simulink model "VIM"  (R2022b)
settings: Solver=ode45  StartTime=0.0  StopTime=1  RelTol=1e-3
PreLoadFcn:
  | % Define motor parameters
  | params.Rs = 0.435;
  | params.Rr = 0.816;
  | params.Ls = 0.006;
  | params.Lr = 0.006;
  | params.Lm = 0.006;
  | params.Xls = 0.006;
  | params.Xlr = 0.006;
  | params.omega_r = 314;
  | params.omega_s = 314;
  | params.dt = 1e-4;
model workspace (MAT data in the model file):
  Lm = Simulink.Parameter
  Lm.Value = 0.006
  Lm.DataType = 'auto'
  Lm.Complexity = 'real'
  Lm.Dimensions = [1 1]
  Lr = Simulink.Parameter
  Lr.Value = 0.006
  Lr.DataType = 'auto'
  Lr.Complexity = 'real'
  Lr.Dimensions = [1 1]
  Ls = Simulink.Parameter
  Ls.Value = 0.006
  Ls.DataType = 'auto'
  Ls.Complexity = 'real'
  Ls.Dimensions = [1 1]
  Rr = Simulink.Parameter
  Rr.Value = 0.816
  Rr.DataType = 'auto'
  Rr.Complexity = 'real'
  Rr.Dimensions = [1 1]
  Rs = Simulink.Parameter
  Rs.Value = 0.435
  Rs.DataType = 'auto'
  Rs.Complexity = 'real'
  Rs.Dimensions = [1 1]
  Sig = Simulink.Signal
  Sig.DataType = 'auto'
  Sig.Dimensions = -1
  Sig.DimensionsMode = 'auto'
  Sig.Complexity = 'auto'
  Sig.SampleTime = -1
  Sig.SamplingMode = 'auto'
  Xlr = Simulink.Parameter
  Xlr.Value = 0.006
  Xlr.DataType = 'auto'
  Xlr.Complexity = 'real'
  Xlr.Dimensions = [1 1]
  Xls = Simulink.Parameter
  Xls.Value = 0.006
  Xls.DataType = 'auto'
  Xls.Complexity = 'real'
  Xls.Dimensions = [1 1]
  dt = Simulink.Parameter
  dt.Value = 0.0001
  dt.DataType = 'auto'
  dt.Complexity = 'real'
  dt.Dimensions = [1 1]
  omega_r = Simulink.Parameter
  omega_r.Value = 314
  omega_r.DataType = 'auto'
  omega_r.Complexity = 'real'
  omega_r.Dimensions = [1 1]
  omega_s = Simulink.Parameter
  omega_s.Value = 314
  omega_s.DataType = 'auto'
  omega_s.Complexity = 'real'
  omega_s.Dimensions = [1 1]
undefined symbols (not defined in the file or in its folder): D1, lagging, motorParams, params_struct_torque, pulse
libraries: slpidlib x4, spsabctodq0Lib x4, spsPLL3phLib x1, spsPulseGeneratorThyristor6PulseLib x1, spsdq0toabcLib x1, spspowerguiLib x1
settings Model: Creator=Dong  LastModifiedBy=Dong

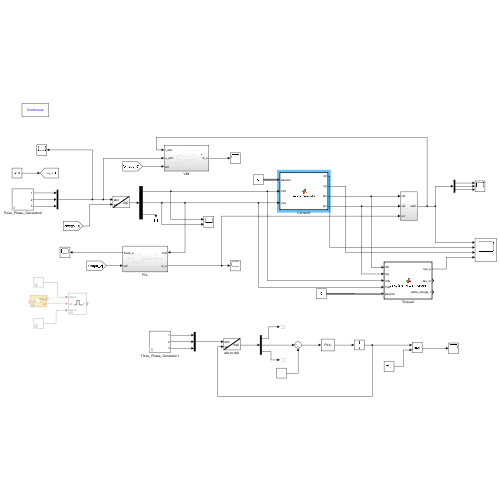
[thumbnail: Simulink's stored preview of the top-level diagram]
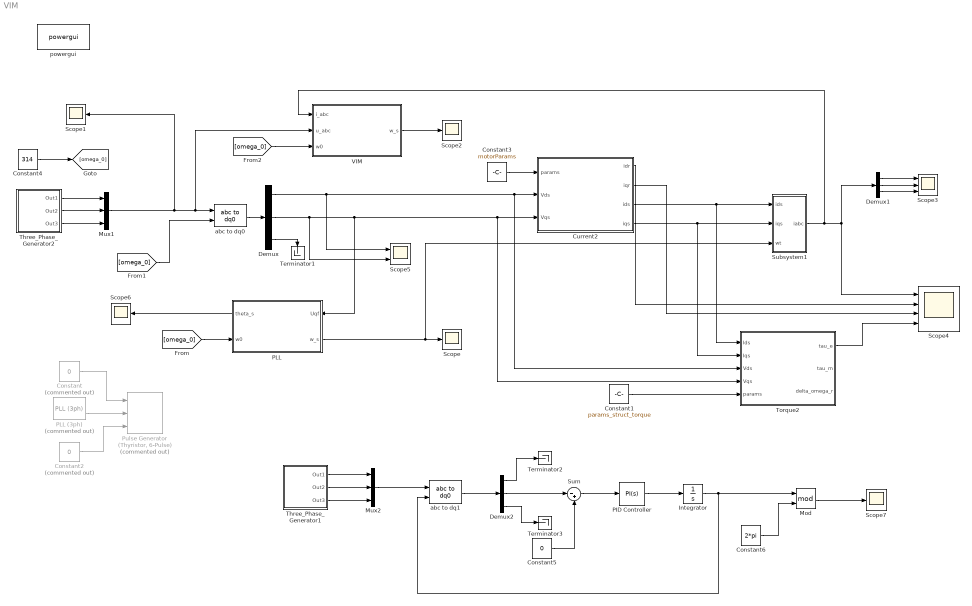
== system VIM ==
  Constant : Constant  Commented=on  Value=0
  Constant1 : Constant  Value=params_struct_torque  OutDataTypeStr=Bus: paramsBusTorque
  Constant2 : Constant  Commented=on  Value=0
  Constant3 : Constant  Value=motorParams  OutDataTypeStr=Bus: motorParamsBus
  Constant4 : Constant  Value=314
  Constant5 : Constant  Value=0
  Constant6 : Constant  Value=2*pi
  Current2 : MATLAB Function  TreatAsAtomicUnit=on
  Demux : Demux  Outputs=3
  Demux1 : Demux  Outputs=3
  Demux2 : Demux  Outputs=3
  Integrator : Integrator
  Mod : Math  Operator=mod
  Mux1 : Mux  Inputs=3
  Mux2 : Mux  Inputs=3
  PID Controller : slpidlib/PID Controller  Controller=PI  Form=Parallel  TimeDomain=Continuous-time  UseExternalTs=off  SampleTime=-1  IntegratorMethod=Forward Euler  FilterMethod=Forward Euler  ControllerParametersSource=internal  P=70  I=2500  UseKiTs=off  D=0  N=100  UseFilter=on  TunerSelectOption=Transfer Function Based (PID Tuner App)  InitialConditionSource=internal  InitialConditionForIntegrator=0  InitialConditionForFilter=0  DifferentiatorICPrevScaledInput=0  ExternalReset=none  TrackingMode=off  Kt=1  LimitOutput=off  SatLimitsSource=internal  UpperSaturationLimit=inf  LowerSaturationLimit=-inf  LinearizeAsGain=on  AntiWindupMode=none  Kb=1  LimitIntegrator=off  UpperIntegratorSaturationLimit=inf  LowerIntegratorSaturationLimit=-inf  POutMin=[]  POutMax=[]  IOutMin=[]  IOutMax=[]  DOutMin=[]  DOutMax=[]  NOutMin=[]  NOutMax=[]  SumOutMin=[]  SumOutMax=[]  SaturationOutMin=[]  SaturationOutMax=[]  PParamMin=[]  PParamMax=[]  IParamMin=[]  IParamMax=[]  DParamMin=[]  DParamMax=[]  NParamMin=[]  NParamMax=[]  KbParamMin=[]  KbParamMax=[]  KtParamMin=[]  KtParamMax=[]  KbOutMin=[]  KbOutMax=[]  KtOutMin=[]  KtOutMax=[]  IntegratorOutMin=[]  IntegratorOutMax=[]  FilterOutMin=[]  FilterOutMax=[]  SumI1OutMin=[]  SumI1OutMax=[]  SumI2OutMin=[]  SumI2OutMax=[]  SumI3OutMin=[]  SumI3OutMax=[]  SumI4OutMin=[]  SumI4OutMax=[]  SumDOutMin=[]  SumDOutMax=[]  DifferentiatorOutMin=[]  DifferentiatorOutMax=[]  FilterDiffOutCoefMin=[]  FilterDiffOutCoefMax=[]  ReciprocalOutMin=[]  ReciprocalOutMax=[]  SumDenOutMin=[]  SumDenOutMax=[]  SumNumOutMin=[]  SumNumOutMax=[]  DivideOutMin=[]  DivideOutMax=[]  UdiffTsProdOutMin=[]  UdiffTsProdOutMax=[]  NTsProdOutMin=[]  NTsProdOutMax=[]  UintegralTsProdOutMin=[]  UintegralTsProdOutMax=[]  UngainTsProdOutMin=[]  UngainTsProdOutMax=[]  ClampingZeroOutDataTypeStr=Inherit: Inherit via back propagation  ClampingZeroOutMin=[]  ClampingZeroOutMax=[]  FilterDenConstantOutDataTypeStr=Inherit: Inherit via back propagation  FilterDenConstantOutMin=[]  FilterDenConstantOutMax=[]  PCopyOutDataTypeStr=Inherit: Inherit via back propagation  PCopyOutMin=[]  PCopyOutMax=[]  NCopyOutDataTypeStr=Inherit: Inherit via back propagation  NCopyOutMin=[]  NCopyOutMax=[]  IntegratorContinuousStateAttributes=''  IntegratorStateMustResolveToSignalObject=off  IntegratorRTWStateStorageClass=Auto  FilterContinuousStateAttributes=''  FilterStateMustResolveToSignalObject=off  FilterRTWStateStorageClass=Auto  ParallelPVariant=InternalParameters  IdealPVariant=Disabled  IVariant=InternalParameters  DVariant=Disabled  IntegratorVariant=Continuous  SatVariant=Disabled  AWVariant=Passthrough  PCopyVariant=Disabled  TRVariant=Disabled  FdbkBlocksVariant=Forward  IdealPFdbkVariant=Disabled  SatFdbkVariant=Disabled  DerivativeFilterVariant=Disabled  NVariant=Disabled  NCopyVariant=Disabled_SignalSpec  FilterICVariant=Disabled  IntegratorICVariant=InternalICs  ExternalResetVariant=Disabled  TRSumVariant=Passthrough  SumFdbkVariant=Disabled  SumVariant=Sum_PI  TsampFilterVariant=InternalTs  TsampNgainVariant=Passthrough  TsampIntegralVariant=Passthrough  ExternalSaturationOutDataTypeStr=Inherit: Same as second input
  PLL : Subsystem
      settings: PortSchema="{\"entries\":[{\"content\":{\"sides\":[{\"content\":{\"connectorIds\":[\"Out2\",\"In1\"]},\"type\":\"ConnectorPlacement.EquallySpacedRectSide\",\"uuid\":\"af5f83a4-7527-4799-92d3-33395b605044\"},{\"content\":{\"connectorIds\":[\"In2\",\"Out1\"],\"side\":\"RIGHT\"},\"type\":\"ConnectorPlacement.EquallySpacedRectSide\",\"uuid\":\"36de21ae-8d82-4c7b-9387-ed93b71e64bb\"},{\"content\":{\"connectorIds\":[],\"side\":\"TOP\"},\"type\":\"ConnectorPlacement.EquallySpacedRectSide\",\"uuid\":\"440d0f6f-e820-4256-be94-60c050b455d0\"}]},\"type\":\"ConnectorPlacement.EquallySpacedConnector\",\"uuid\":\"20572b40-4a5f-41c5-8c6b-bc5bfa0c4be0\"}],\"packageUris\":[\"http://schema.mathworks.com/mf0/Connector/R2020b\"],\"version\":\"1.0\"}"
  PLL (3ph) : spsPLL3phLib/PLL (3ph)  Commented=on  Fmin=49  Par_Init=[0, 50]  ParK=[180, 3200, 1]  TcD=1e-4  MaxRateChangeFreq=12  FilterCutOffFreq=25  Ts=0  AGC=on
  "Pulse Generator (Thyristor, 6-Pulse)" : spsPulseGeneratorThyristor6PulseLib/Pulse Generator (Thyristor, 6-Pulse)  Commented=on  GenType=6-pulse  Delta=D1 (lagging)  pwidth=60  Double_Pulse=off  Ts=0
      settings: LibrarySourceBlock=|
      | sps_lib/Power Electronics/Power Electronics Control/Pulse Generator
      | (Thyristor, 6-Pulse)
  Scope{,1..2,6..7} (5 alike) : Scope
  Scope3 : Scope  NumInputPorts=3
  Scope4 : Scope  NumInputPorts=4
  Scope5 : Scope  NumInputPorts=2
  Subsystem1 : Subsystem
  Sum : Sum  Inputs=|-+
  Terminator1 : Terminator
  Terminator2 : Terminator
  Terminator3 : Terminator
  Three_Phase_Generator1 : Subsystem  mask{freq=50, alpha=120, amplitude=240}
      mask prompts: freq "Frequenz"; alpha "Pahse"
      mask DialogControl ParameterGroupVar Prompt: 参数
  Three_Phase_Generator2 : Subsystem  mask{freq=50, alpha=120, amplitude=240}
      mask prompts: freq "Frequenz"; alpha "Pahse"
      mask DialogControl ParameterGroupVar Prompt: 参数
  Torque2 : MATLAB Function  TreatAsAtomicUnit=on
  VIM : Subsystem
  abc to dq0 : spsabctodq0Lib/abc to dq0  Alignment=90 degrees behind phase A axis
  abc to dq1 : spsabctodq0Lib/abc to dq0  Alignment=90 degrees behind phase A axis
  powergui : spspowerguiLib/powergui  Priority=1  SimulationMode=Continuous  SampleTime=50e-6  frequency=60  Iterations=50  frequencyindice=60  Pbase=100e6  ErrMax=1e-4  UnitsV=kV  UnitsW=MW  buscounter=0  FunctionMessages=off  echomessages=off  EnableUseOfTLC=off  CurrentSourceSwitches=off  DisableSnubberDevices=off  DisableRonSwitches=off  DisableVfSwitches=off  DisplayEquations=off  AutomaticDiscreteSolvers=off  SolverType=Tustin/Backward Euler (TBE)  Interpol=off  ExternalGateDelay=off  methode=off  Ts=100  x0status=blocks  SPID=on  SwTol=0  HookPort=off  NonlinearTolerance=1e-4  nMaxIteration=100  ContinueOnMaxIteration=off  RestoreLinks=warning  ResistiveCurrentMeasurement=off  Frange=[0:2:500]  Ylog=off  Xlog=on  ShowGrid=off  save=off  variable=ZData  structure=0  ZoomFFT=off  StartTime=0.0  cycles=1  DisplayStyle=1  fundamental=60  FreqAxis=off  MaxFrequency=1000  frequencyindicesteady=1  RmsSteady=1  display=off
  wires:
  Mux1/1 -> Scope1/1, abc to dq0/1, VIM/2(u_abc)
  abc to dq0/1 -> Demux/1
  Constant1/1 -> Torque2/5(params)
  Constant3/1 -> Current2/1(params)
  Demux/3 -> Terminator1/1
  Current2/3(ids) -> Torque2/1(Ids), Subsystem1/1(ids)
  Current2/4(iqs) -> Torque2/2(Iqs), Subsystem1/2(iqs)
  Demux/1 -> Scope5/1, Current2/2(Vds), Torque2/3(Vds)
  PLL/1(w_s) -> Scope/1, Subsystem1/3(wt)
  VIM/1(w_s) -> Scope2/1
  Torque2/1(tau_e) -> Scope4/4
  Current2/2(iqr) -> Scope4/3
  Current2/1(idr) -> Scope4/2
  Subsystem1/1(iabc) -> VIM/1(i_abc), Scope4/1, Demux1/1
  Demux/2 -> Scope5/2, Torque2/4(Vqs), Current2/3(Vqs), PLL/2(Uqf)
  Demux1/1 -> Scope3/1
  Demux1/2 -> Scope3/2
  Demux1/3 -> Scope3/3
  Three_Phase_Generator2/1(Out1) -> Mux1/1
  Three_Phase_Generator2/2(Out2) -> Mux1/2
  Three_Phase_Generator2/3(Out3) -> Mux1/3
  Constant4/1 -> [omega_0]
  [omega_0] -> PLL/1(w0)
  PLL/2(theta_s) -> Scope6/1
  [omega_0] -> VIM/3(w0)
  [omega_0] -> abc to dq0/2
  PLL (3ph)/2 -> "Pulse Generator (Thyristor, 6-Pulse)"/2
  Constant/1 -> "Pulse Generator (Thyristor, 6-Pulse)"/1
  Constant2/1 -> "Pulse Generator (Thyristor, 6-Pulse)"/3
  Three_Phase_Generator1/3(Out3) -> Mux2/3
  Three_Phase_Generator1/2(Out2) -> Mux2/2
  Three_Phase_Generator1/1(Out1) -> Mux2/1
  Mux2/1 -> abc to dq1/1
  abc to dq1/1 -> Demux2/1
  Demux2/1 -> Terminator2/1
  Demux2/3 -> Terminator3/1
  Constant5/1 -> Sum/2
  Sum/1 -> PID Controller/1
  PID Controller/1 -> Integrator/1
  Integrator/1 -> Mod/1, abc to dq1/2
  Demux2/2 -> Sum/1
  Constant6/1 -> Mod/2
  Mod/1 -> Scope7/1

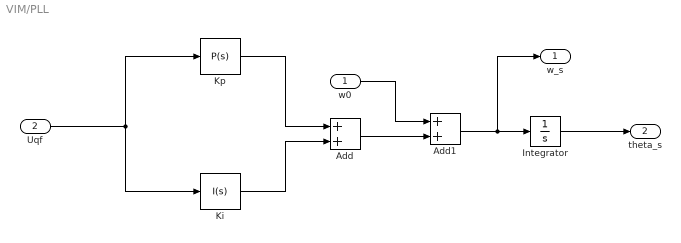
== system VIM/PLL ==
  w0 : Inport
  Uqf : Inport  Port=2
  Add : Sum
  Add1 : Sum
  Integrator : Integrator
  Ki : slpidlib/PID Controller  Controller=I  Form=Parallel  TimeDomain=Continuous-time  UseExternalTs=off  SampleTime=-1  IntegratorMethod=Forward Euler  FilterMethod=Forward Euler  ControllerParametersSource=internal  P=1  I=5  UseKiTs=off  D=0  N=100  UseFilter=on  TunerSelectOption=Transfer Function Based (PID Tuner App)  InitialConditionSource=internal  InitialConditionForIntegrator=0  InitialConditionForFilter=0  DifferentiatorICPrevScaledInput=0  ExternalReset=none  TrackingMode=off  Kt=1  LimitOutput=off  SatLimitsSource=internal  UpperSaturationLimit=inf  LowerSaturationLimit=-inf  LinearizeAsGain=on  AntiWindupMode=none  Kb=1  LimitIntegrator=off  UpperIntegratorSaturationLimit=inf  LowerIntegratorSaturationLimit=-inf  POutMin=[]  POutMax=[]  IOutMin=[]  IOutMax=[]  DOutMin=[]  DOutMax=[]  NOutMin=[]  NOutMax=[]  SumOutMin=[]  SumOutMax=[]  SaturationOutMin=[]  SaturationOutMax=[]  PParamMin=[]  PParamMax=[]  IParamMin=[]  IParamMax=[]  DParamMin=[]  DParamMax=[]  NParamMin=[]  NParamMax=[]  KbParamMin=[]  KbParamMax=[]  KtParamMin=[]  KtParamMax=[]  KbOutMin=[]  KbOutMax=[]  KtOutMin=[]  KtOutMax=[]  IntegratorOutMin=[]  IntegratorOutMax=[]  FilterOutMin=[]  FilterOutMax=[]  SumI1OutMin=[]  SumI1OutMax=[]  SumI2OutMin=[]  SumI2OutMax=[]  SumI3OutMin=[]  SumI3OutMax=[]  SumI4OutMin=[]  SumI4OutMax=[]  SumDOutMin=[]  SumDOutMax=[]  DifferentiatorOutMin=[]  DifferentiatorOutMax=[]  FilterDiffOutCoefMin=[]  FilterDiffOutCoefMax=[]  ReciprocalOutMin=[]  ReciprocalOutMax=[]  SumDenOutMin=[]  SumDenOutMax=[]  SumNumOutMin=[]  SumNumOutMax=[]  DivideOutMin=[]  DivideOutMax=[]  UdiffTsProdOutMin=[]  UdiffTsProdOutMax=[]  NTsProdOutMin=[]  NTsProdOutMax=[]  UintegralTsProdOutMin=[]  UintegralTsProdOutMax=[]  UngainTsProdOutMin=[]  UngainTsProdOutMax=[]  ClampingZeroOutDataTypeStr=Inherit: Inherit via back propagation  ClampingZeroOutMin=[]  ClampingZeroOutMax=[]  FilterDenConstantOutDataTypeStr=Inherit: Inherit via back propagation  FilterDenConstantOutMin=[]  FilterDenConstantOutMax=[]  PCopyOutDataTypeStr=Inherit: Inherit via back propagation  PCopyOutMin=[]  PCopyOutMax=[]  NCopyOutDataTypeStr=Inherit: Inherit via back propagation  NCopyOutMin=[]  NCopyOutMax=[]  IntegratorContinuousStateAttributes=''  IntegratorStateMustResolveToSignalObject=off  IntegratorRTWStateStorageClass=Auto  FilterContinuousStateAttributes=''  FilterStateMustResolveToSignalObject=off  FilterRTWStateStorageClass=Auto  ParallelPVariant=Disabled  IdealPVariant=Disabled  IVariant=InternalParameters  DVariant=Disabled  IntegratorVariant=Continuous  SatVariant=Disabled  AWVariant=Passthrough  PCopyVariant=Disabled  TRVariant=Disabled  FdbkBlocksVariant=Forward  IdealPFdbkVariant=Disabled  SatFdbkVariant=Disabled  DerivativeFilterVariant=Disabled  NVariant=Disabled  NCopyVariant=Disabled_SignalSpec  FilterICVariant=Disabled  IntegratorICVariant=InternalICs  ExternalResetVariant=Disabled  TRSumVariant=Passthrough  SumFdbkVariant=Disabled  SumVariant=Passthrough_I  TsampFilterVariant=InternalTs  TsampNgainVariant=Passthrough  TsampIntegralVariant=Passthrough  ExternalSaturationOutDataTypeStr=Inherit: Same as second input
  Kp : slpidlib/PID Controller  Controller=P  Form=Parallel  TimeDomain=Continuous-time  UseExternalTs=off  SampleTime=-1  IntegratorMethod=Forward Euler  FilterMethod=Forward Euler  ControllerParametersSource=internal  P=7  I=1  UseKiTs=off  D=0  N=100  UseFilter=on  TunerSelectOption=Transfer Function Based (PID Tuner App)  InitialConditionSource=internal  InitialConditionForIntegrator=0  InitialConditionForFilter=0  DifferentiatorICPrevScaledInput=0  ExternalReset=none  TrackingMode=off  Kt=1  LimitOutput=off  SatLimitsSource=internal  UpperSaturationLimit=inf  LowerSaturationLimit=-inf  LinearizeAsGain=on  AntiWindupMode=none  Kb=1  LimitIntegrator=off  UpperIntegratorSaturationLimit=inf  LowerIntegratorSaturationLimit=-inf  POutMin=[]  POutMax=[]  IOutMin=[]  IOutMax=[]  DOutMin=[]  DOutMax=[]  NOutMin=[]  NOutMax=[]  SumOutMin=[]  SumOutMax=[]  SaturationOutMin=[]  SaturationOutMax=[]  PParamMin=[]  PParamMax=[]  IParamMin=[]  IParamMax=[]  DParamMin=[]  DParamMax=[]  NParamMin=[]  NParamMax=[]  KbParamMin=[]  KbParamMax=[]  KtParamMin=[]  KtParamMax=[]  KbOutMin=[]  KbOutMax=[]  KtOutMin=[]  KtOutMax=[]  IntegratorOutMin=[]  IntegratorOutMax=[]  FilterOutMin=[]  FilterOutMax=[]  SumI1OutMin=[]  SumI1OutMax=[]  SumI2OutMin=[]  SumI2OutMax=[]  SumI3OutMin=[]  SumI3OutMax=[]  SumI4OutMin=[]  SumI4OutMax=[]  SumDOutMin=[]  SumDOutMax=[]  DifferentiatorOutMin=[]  DifferentiatorOutMax=[]  FilterDiffOutCoefMin=[]  FilterDiffOutCoefMax=[]  ReciprocalOutMin=[]  ReciprocalOutMax=[]  SumDenOutMin=[]  SumDenOutMax=[]  SumNumOutMin=[]  SumNumOutMax=[]  DivideOutMin=[]  DivideOutMax=[]  UdiffTsProdOutMin=[]  UdiffTsProdOutMax=[]  NTsProdOutMin=[]  NTsProdOutMax=[]  UintegralTsProdOutMin=[]  UintegralTsProdOutMax=[]  UngainTsProdOutMin=[]  UngainTsProdOutMax=[]  ClampingZeroOutDataTypeStr=Inherit: Inherit via back propagation  ClampingZeroOutMin=[]  ClampingZeroOutMax=[]  FilterDenConstantOutDataTypeStr=Inherit: Inherit via back propagation  FilterDenConstantOutMin=[]  FilterDenConstantOutMax=[]  PCopyOutDataTypeStr=Inherit: Inherit via back propagation  PCopyOutMin=[]  PCopyOutMax=[]  NCopyOutDataTypeStr=Inherit: Inherit via back propagation  NCopyOutMin=[]  NCopyOutMax=[]  IntegratorContinuousStateAttributes=''  IntegratorStateMustResolveToSignalObject=off  IntegratorRTWStateStorageClass=Auto  FilterContinuousStateAttributes=''  FilterStateMustResolveToSignalObject=off  FilterRTWStateStorageClass=Auto  ParallelPVariant=InternalParameters  IdealPVariant=Disabled  IVariant=Disabled  DVariant=Disabled  IntegratorVariant=Disabled  SatVariant=Disabled  AWVariant=Disabled  PCopyVariant=Disabled  TRVariant=Disabled  FdbkBlocksVariant=Forward  IdealPFdbkVariant=Disabled  SatFdbkVariant=Disabled  DerivativeFilterVariant=Disabled  NVariant=Disabled  NCopyVariant=Disabled_SignalSpec  FilterICVariant=Disabled  IntegratorICVariant=Disabled  ExternalResetVariant=Disabled  TRSumVariant=Passthrough  SumFdbkVariant=Disabled  SumVariant=Passthrough_P  TsampFilterVariant=InternalTs  TsampNgainVariant=Passthrough  TsampIntegralVariant=Disabled_SignalSpec  ExternalSaturationOutDataTypeStr=Inherit: Same as second input
  w_s : Outport
  theta_s : Outport  Port=2
  wires:
  Uqf/1 -> Kp/1, Ki/1
  Kp/1 -> Add/1
  Ki/1 -> Add/2
  Add/1 -> Add1/2
  w0/1 -> Add1/1
  Add1/1 -> w_s/1, Integrator/1
  Integrator/1 -> theta_s/1

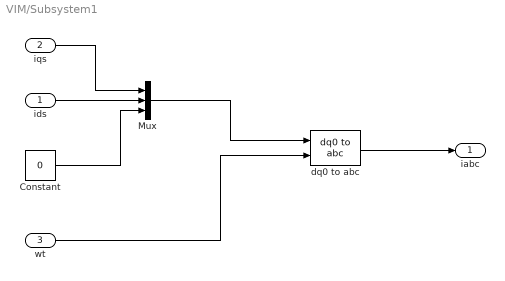
== system VIM/Subsystem1 ==
  ids : Inport
  iqs : Inport  Port=2
  wt : Inport  Port=3
  Constant : Constant  Value=0
  Mux : Mux  Inputs=3
  dq0 to abc : spsdq0toabcLib/dq0 to abc  Alignment=90 degrees behind phase A axis
  iabc : Outport
  wires:
  dq0 to abc/1 -> iabc/1
  wt/1 -> dq0 to abc/2
  Mux/1 -> dq0 to abc/1
  iqs/1 -> Mux/1
  ids/1 -> Mux/2
  Constant/1 -> Mux/3

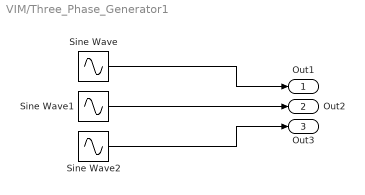
== system VIM/Three_Phase_Generator1 ==
  Sine Wave : Sin  Amplitude=amplitude  Frequency=freq*2*pi  Phase=0*alpha/180*pi  SampleTime=0
  Sine Wave1 : Sin  Amplitude=amplitude  Frequency=freq*2*pi  Phase=1*alpha/180*pi  SampleTime=0
  Sine Wave2 : Sin  Amplitude=amplitude  Frequency=freq*2*pi  Phase=2*alpha/180*pi  SampleTime=0
  Out1 : Outport
  Out2 : Outport  Port=2
  Out3 : Outport  Port=3
  wires:
  Sine Wave1/1 -> Out2/1
  Sine Wave/1 -> Out1/1
  Sine Wave2/1 -> Out3/1

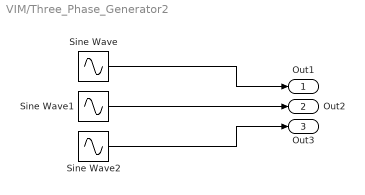
== system VIM/Three_Phase_Generator2 ==
  Sine Wave : Sin  Amplitude=amplitude  Frequency=freq*2*pi  Phase=0*alpha/180*pi  SampleTime=0
  Sine Wave1 : Sin  Amplitude=amplitude  Frequency=freq*2*pi  Phase=1*alpha/180*pi  SampleTime=0
  Sine Wave2 : Sin  Amplitude=amplitude  Frequency=freq*2*pi  Phase=2*alpha/180*pi  SampleTime=0
  Out1 : Outport
  Out2 : Outport  Port=2
  Out3 : Outport  Port=3
  wires:
  Sine Wave2/1 -> Out3/1
  Sine Wave/1 -> Out1/1
  Sine Wave1/1 -> Out2/1

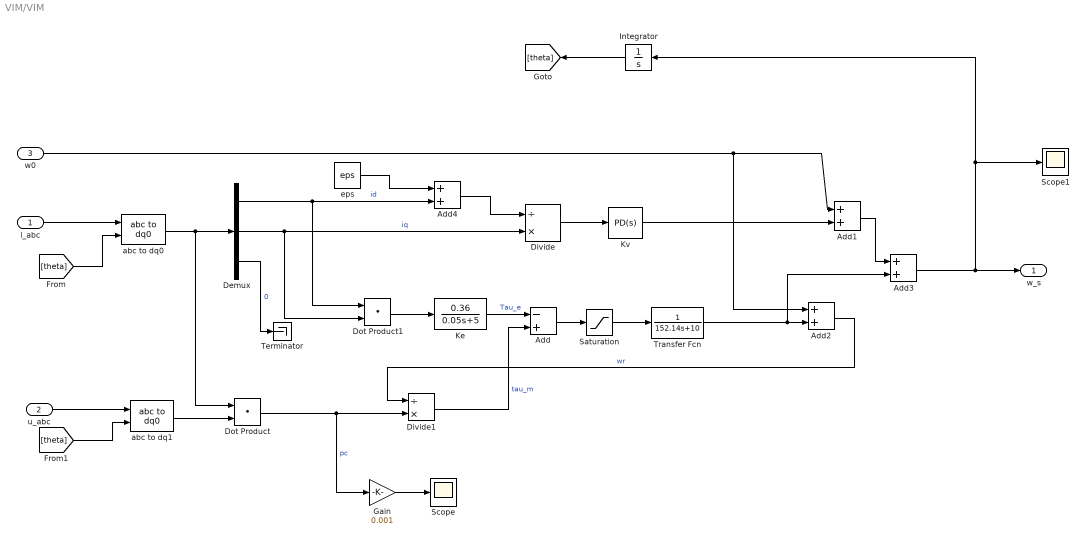
== system VIM/VIM ==
  i_abc : Inport
  u_abc : Inport  Port=2
  w0 : Inport  Port=3
  Add : Sum  Inputs=-+
  Add{1..4} (4 alike) : Sum
  Demux : Demux  Outputs=3
  Divide : Product  Inputs=/*
  Divide1 : Product  Inputs=/*
  Dot Product : DotProduct  OutDataTypeStr=Inherit: Inherit via internal rule
  Dot Product1 : DotProduct  OutDataTypeStr=Inherit: Inherit via internal rule
  Gain : Gain  Gain=0.001
  Integrator : Integrator
  Ke : TransferFcn  Numerator=[0.36]  Denominator=[0.05 5]  ParameterTunability=Optimized
  Kv : slpidlib/PID Controller  Controller=PD  Form=Parallel  TimeDomain=Continuous-time  UseExternalTs=off  SampleTime=-1  IntegratorMethod=Forward Euler  FilterMethod=Forward Euler  ControllerParametersSource=internal  P=0.01  I=1  UseKiTs=off  D=1  N=100  UseFilter=on  TunerSelectOption=Transfer Function Based (PID Tuner App)  InitialConditionSource=internal  InitialConditionForIntegrator=0  InitialConditionForFilter=0  DifferentiatorICPrevScaledInput=0  ExternalReset=none  TrackingMode=off  Kt=1  LimitOutput=off  SatLimitsSource=internal  UpperSaturationLimit=inf  LowerSaturationLimit=-inf  LinearizeAsGain=on  AntiWindupMode=none  Kb=1  LimitIntegrator=off  UpperIntegratorSaturationLimit=inf  LowerIntegratorSaturationLimit=-inf  POutMin=[]  POutMax=[]  IOutMin=[]  IOutMax=[]  DOutMin=[]  DOutMax=[]  NOutMin=[]  NOutMax=[]  SumOutMin=[]  SumOutMax=[]  SaturationOutMin=[]  SaturationOutMax=[]  PParamMin=[]  PParamMax=[]  IParamMin=[]  IParamMax=[]  DParamMin=[]  DParamMax=[]  NParamMin=[]  NParamMax=[]  KbParamMin=[]  KbParamMax=[]  KtParamMin=[]  KtParamMax=[]  KbOutMin=[]  KbOutMax=[]  KtOutMin=[]  KtOutMax=[]  IntegratorOutMin=[]  IntegratorOutMax=[]  FilterOutMin=[]  FilterOutMax=[]  SumI1OutMin=[]  SumI1OutMax=[]  SumI2OutMin=[]  SumI2OutMax=[]  SumI3OutMin=[]  SumI3OutMax=[]  SumI4OutMin=[]  SumI4OutMax=[]  SumDOutMin=[]  SumDOutMax=[]  DifferentiatorOutMin=[]  DifferentiatorOutMax=[]  FilterDiffOutCoefMin=[]  FilterDiffOutCoefMax=[]  ReciprocalOutMin=[]  ReciprocalOutMax=[]  SumDenOutMin=[]  SumDenOutMax=[]  SumNumOutMin=[]  SumNumOutMax=[]  DivideOutMin=[]  DivideOutMax=[]  UdiffTsProdOutMin=[]  UdiffTsProdOutMax=[]  NTsProdOutMin=[]  NTsProdOutMax=[]  UintegralTsProdOutMin=[]  UintegralTsProdOutMax=[]  UngainTsProdOutMin=[]  UngainTsProdOutMax=[]  ClampingZeroOutDataTypeStr=Inherit: Inherit via back propagation  ClampingZeroOutMin=[]  ClampingZeroOutMax=[]  FilterDenConstantOutDataTypeStr=Inherit: Inherit via back propagation  FilterDenConstantOutMin=[]  FilterDenConstantOutMax=[]  PCopyOutDataTypeStr=Inherit: Inherit via back propagation  PCopyOutMin=[]  PCopyOutMax=[]  NCopyOutDataTypeStr=Inherit: Inherit via back propagation  NCopyOutMin=[]  NCopyOutMax=[]  IntegratorContinuousStateAttributes=''  IntegratorStateMustResolveToSignalObject=off  IntegratorRTWStateStorageClass=Auto  FilterContinuousStateAttributes=''  FilterStateMustResolveToSignalObject=off  FilterRTWStateStorageClass=Auto  ParallelPVariant=InternalParameters  IdealPVariant=Disabled  IVariant=Disabled  DVariant=InternalParameters  IntegratorVariant=Disabled  SatVariant=Disabled  AWVariant=Disabled  PCopyVariant=Disabled  TRVariant=Disabled  FdbkBlocksVariant=Forward  IdealPFdbkVariant=Disabled  SatFdbkVariant=Disabled  DerivativeFilterVariant=ContFilter  NVariant=InternalParameters  NCopyVariant=Disabled  FilterICVariant=InternalICsFilter  IntegratorICVariant=Disabled  ExternalResetVariant=Disabled  TRSumVariant=Passthrough  SumFdbkVariant=Disabled  SumVariant=Sum_PD  TsampFilterVariant=InternalTs  TsampNgainVariant=Passthrough  TsampIntegralVariant=Disabled_SignalSpec  ExternalSaturationOutDataTypeStr=Inherit: Same as second input
  Saturation : Saturate  UpperLimit=1  LowerLimit=-1
  Scope : Scope
  Scope1 : Scope
  Terminator : Terminator
  Transfer Fcn : TransferFcn  Denominator=[152.14 10]  ParameterTunability=Optimized
  abc to dq0 : spsabctodq0Lib/abc to dq0  Alignment=90 degrees behind phase A axis
  abc to dq1 : spsabctodq0Lib/abc to dq0  Alignment=90 degrees behind phase A axis
  eps : Constant  Value=eps
  w_s : Outport
  wires:
  i_abc/1 -> abc to dq0/1
  u_abc/1 -> abc to dq1/1
  abc to dq1/1 -> Dot Product/2
  abc to dq0/1 -> Dot Product/1, Demux/1
  Demux/1 -> Dot Product1/1, Add4/2  "id"
  Demux/2 -> Dot Product1/2, Divide/2  "iq"
  Divide/1 -> Kv/1
  Kv/1 -> Add1/2
  w0/1 -> Add2/1, Add1/1
  Dot Product1/1 -> Ke/1
  Divide1/1 -> Add/2  "tau_m"
  Add/1 -> Saturation/1
  Transfer Fcn/1 -> Add3/2, Add2/2
  Add1/1 -> Add3/1
  Add3/1 -> w_s/1, Scope1/1, Integrator/1
  Integrator/1 -> [theta]
  [theta] -> abc to dq1/2
  [theta] -> abc to dq0/2
  Demux/3 -> Terminator/1  "0"
  Dot Product/1 -> Divide1/2, Gain/1  "pc"
  Ke/1 -> Add/1  "Tau_e"
  Saturation/1 -> Transfer Fcn/1
  eps/1 -> Add4/1
  Add4/1 -> Divide/1
  Gain/1 -> Scope/1
  Add2/1 -> Divide1/1  "wr"

== matlab function VIM/Torque2 ==
  settings: updateMethod=DISCRETE
  data: Ids input double size=[1 1]; Iqs input double size=[1 1]; Vds input double size=[1 1]; Vqs input double size=[1 1]; tau_e output double size=[1 1]; params input Bus: paramsBusTorque; tau_m output double size=[1 1]; delta_omega_r output double size=[1 1]
function [tau_e, tau_m, delta_omega_r] = calculate_virtual_torque(Ids, Iqs, Vds, Vqs, params)
%#codegen
% Inputs:
% Vds - d-axis stator voltage
% Vqs - q-axis stator voltage
% Ids - d-axis stator current
% Iqs - q-axis stator current
% params - structure containing motor parameters
% Outputs:
% tau_e - electromagnetic torque
% tau_m - mechanical torque
% delta_omega_r - change in rotor angular speed

% Extract parameters from the input structure
%Rs = params.Rs;
Rr = params.Rr;
Ls = params.Ls;
Lr = params.Lr;
Lm = params.Lm;
psi_dr = params.psi_dr;
omega0 = params.omega0;
D = params.D;
J = params.J;
delta_omega_r = params.delta_omega_r;

% Calculate stator flux linkages
psi_ds = (Ls - (Lm^2 / Lr)) * Ids + (Lm / Lr) * psi_dr;
psi_qs = (Ls - (Lm^2 / Lr)) * Iqs;

% Calculate electromagnetic torque
tau_e = (3/2) * (Lm / Lr) * psi_dr * Iqs;

% Calculate mechanical torque
Pc = Vds * Ids + Vqs * Iqs; % Output active power
tau_m = Pc / (omega0 + delta_omega_r);

% Calculate change in rotor angular speed
% Use a first-order system to approximate the dynamics
tau_e_freq = (3/2) * (Rr * Lm^2) / (Rr * Lr) * Ids * Iqs; % Simplified frequency domain torque
delta_omega_r = (1 / (J + D)) * (tau_m - tau_e_freq);

% No need to use impulse or tf functions
end

== matlab function VIM/Current2 ==
  settings: updateMethod=DISCRETE
  data: params input Bus: motorParamsBus; Vds input double size=[1 1]; Vqs input double size=[1 1]; idr output double size=[1 1]; iqr output; ids output double size=[1 1]; iqs output double size=[1 1]
function [idr, iqr, ids, iqs] = motorCurrents(params, Vds, Vqs)
% Inputs:
% Vqs - q-axis stator voltage
% Vds - d-axis stator voltage
% params - structure containing motor parameters
% Outputs:
% ids - d-axis stator current
% iqs - q-axis stator current
% idr - d-axis rotor current
% iqr - q-axis rotor current

% Motor parameters
Rs = params.Rs; % Stator resistance
Rr = params.Rr; % Rotor resistance
Ls = params.Ls; % Stator inductance
Lr = params.Lr; % Rotor inductance
Lm = params.Lm; % Mutual inductance

omega_r = params.omega_r; % Rotor angular velocity
omega_s = params.omega_s; % Synchronous angular velocity

% Initialize state variables
persistent lambda_ds lambda_qs lambda_dr lambda_qr;
if isempty(lambda_ds)
    lambda_ds = 0;
    lambda_qs = 0;
    lambda_dr = 0;
    lambda_qr = 0;
end

% Time step (assumed constant for simplicity)
dt = params.dt;


% Calculate stator and rotor currents
ids = (lambda_ds - Lm * lambda_dr) / Ls;
iqs = (lambda_qs - Lm * lambda_qr) / Ls;
idr = (lambda_dr - Lm * ids) / Lr;
iqr = (lambda_qr - Lm * iqs) / Lr;


% Stator flux linkages
lambda_ds = lambda_ds + (Vds - Rs * ids + omega_r * lambda_qs) * dt;
lambda_qs = lambda_qs + (Vqs - Rs * iqs - omega_r * lambda_ds) * dt;

% Rotor flux linkages
lambda_dr = lambda_dr + (-Rr * idr + (omega_s - omega_r) * lambda_qr) * dt;
lambda_qr = lambda_qr + (-Rr * iqr - (omega_s - omega_r) * lambda_dr) * dt;
